simulink model "bicicle_model"  (R2016b)
settings: Solver=VariableStepAuto  StartTime=0.0  StopTime=10.0  RelTol=1e-3
undefined symbols (not defined in the file): x0
settings Model: Creator=Nexel  LastModifiedBy=Nexel

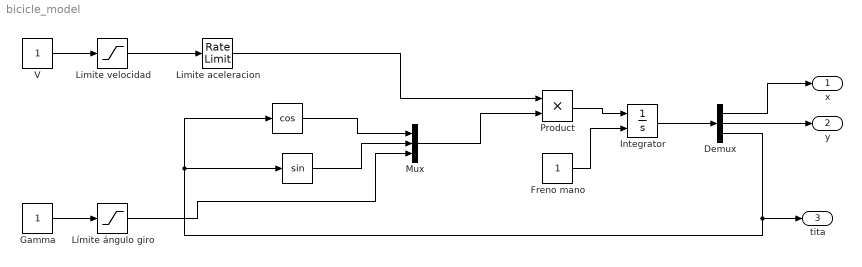
== system bicicle_model ==
  " " : Trigonometry  Operator=cos
  " " : Trigonometry
  Demux : Demux  Outputs=3
  Freno mano : Constant
  "Gamma " : Constant
  Integrator : Integrator  InitialConditionSource=external  InitialCondition=x0
  Limite aceleracion : RateLimiter  SampleTimeMode=inherited
  Limite velocidad : Saturate  UpperLimit=1  LowerLimit=-1
  "Límite ángulo giro " : Saturate  UpperLimit=2  LowerLimit=-2
  Mux : Mux  Inputs=3
  Product : Product
  "V " : Constant
  x : Outport
  y : Outport  Port=2
  tita : Outport  Port=3
  wires:
  "Gamma "/1 -> "Límite ángulo giro "/1
  "V "/1 -> Limite velocidad/1
  Limite velocidad/1 -> Limite aceleracion/1
  Limite aceleracion/1 -> Product/1
  Freno mano/1 -> Integrator/2
  " "/1 -> Mux/1
  " "/1 -> Mux/2
  "Límite ángulo giro "/1 -> Mux/3
  Mux/1 -> Product/2
  Product/1 -> Integrator/1
  Integrator/1 -> Demux/1
  Demux/1 -> x/1
  Demux/2 -> y/1
  Demux/3 -> " "/1, " "/1, tita/1
